simulink model "first_order_separable_diff"  (R2022a)
settings: Solver=VariableStepAuto  StartTime=0.0  StopTime=10.0  RelTol=1e-3
settings Model: Creator=Home computer  LastModifiedBy=Home computer

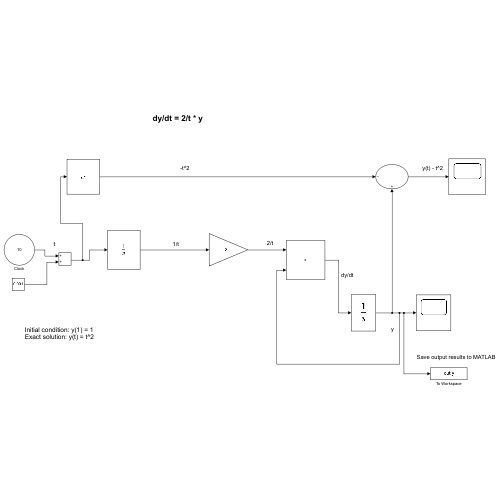
[thumbnail: Simulink's stored preview of the top-level diagram]
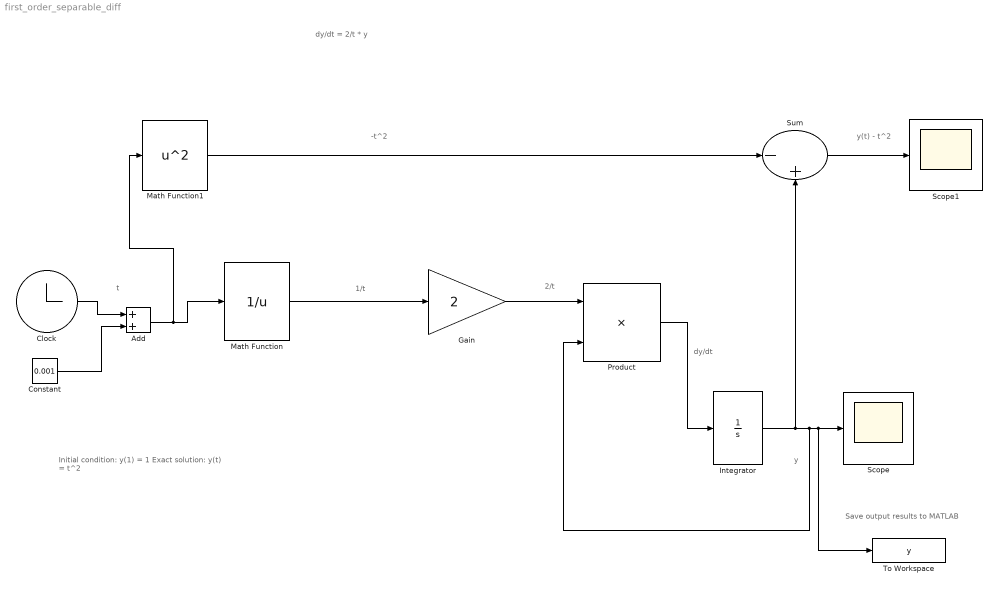
== system first_order_separable_diff ==
  note: Save output results to MATLAB
  note: y(t) - t^2
  note: -t^2
  note: Initial condition: y(1) = 1
      | Exact solution: y(t) = t^2
  note: y
  note: dy/dt = 2/t * y
  note: 2/t
  note: dy/dt
  note: 1/t
  note: t
  Add : Sum
  Clock : Clock
  Constant : Constant  Value=0.001
  Gain : Gain  Gain=2
  Integrator : Integrator  InitialCondition=1
  Math Function : Math  Operator=reciprocal
  Math Function1 : Math  Operator=square
  Product : Product
  Scope : Scope
  Scope1 : Scope
  Sum : Sum  Inputs=|-+
  To Workspace : ToWorkspace  VariableName=y  SaveFormat=Timeseries  SampleTime=-1
  wires:
  Clock/1 -> Add/1
  Math Function/1 -> Gain/1
  Gain/1 -> Product/1
  Product/1 -> Integrator/1
  Integrator/1 -> To Workspace/1, Scope/1, Product/2, Sum/2
  Constant/1 -> Add/2
  Add/1 -> Math Function1/1, Math Function/1
  Math Function1/1 -> Sum/1
  Sum/1 -> Scope1/1
